simulink model "Avionics"  (R2022b)
settings: Solver=VariableStepAuto  StartTime=0.0  StopTime=10.0  RelTol=1e-3
settings Model: Creator=amira  LastModifiedBy=amira

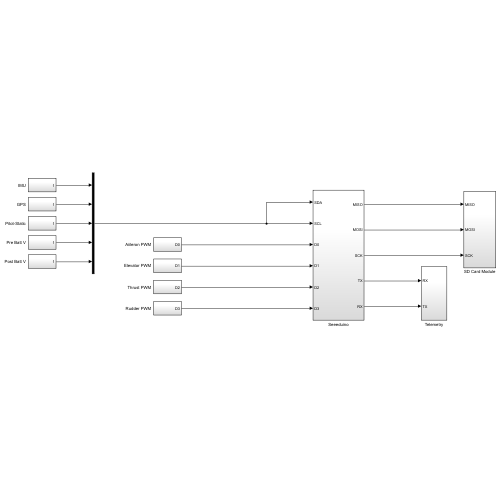
[thumbnail: Simulink's stored preview of the top-level diagram]
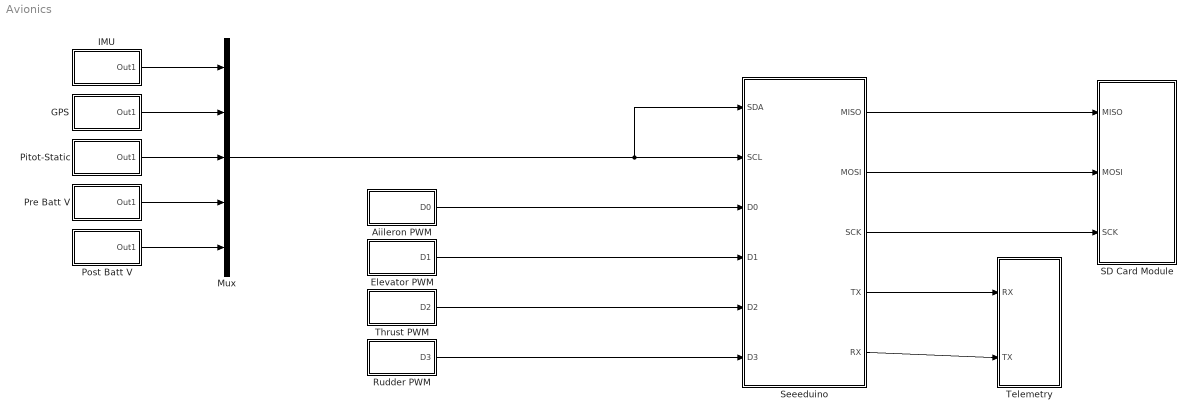
== system Avionics ==
  Aiileron PWM : Subsystem
  Elevator PWM : Subsystem
  GPS : Subsystem
  IMU : Subsystem
  Mux : Mux  Inputs=5
  Pitot-Static : Subsystem
  Post Batt V : Subsystem
  Pre Batt V : Subsystem
  Rudder PWM : Subsystem
  SD Card Module : Subsystem
  Seeeduino : Subsystem
  Telemetry : Subsystem
  Thrust PWM : Subsystem
  wires:
  Pitot-Static/1(Out1) -> Mux/3
  GPS/1(Out1) -> Mux/2
  IMU/1(Out1) -> Mux/1
  Pre Batt V/1(Out1) -> Mux/4
  Post Batt V/1(Out1) -> Mux/5
  Mux/1 -> Seeeduino/1(SDA), Seeeduino/2(SCL)
  Rudder PWM/1(D3) -> Seeeduino/6(D3)
  Thrust PWM/1(D2) -> Seeeduino/5(D2)
  Aiileron PWM/1(D0) -> Seeeduino/3(D0)
  Elevator PWM/1(D1) -> Seeeduino/4(D1)
  Seeeduino/1(MISO) -> SD Card Module/1(MISO)
  Seeeduino/2(MOSI) -> SD Card Module/2(MOSI)
  Seeeduino/3(SCK) -> SD Card Module/3(SCK)
  Seeeduino/4(TX) -> Telemetry/1(RX)
  Seeeduino/5(RX) -> Telemetry/2(TX)

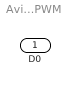
== system Avionics/Aiileron PWM ==
  D0 : Outport

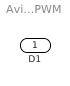
== system Avionics/Elevator PWM ==
  D1 : Outport

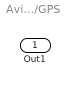
== system Avionics/GPS ==
  Out1 : Outport

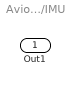
== system Avionics/IMU ==
  Out1 : Outport

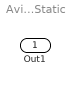
== system Avionics/Pitot-Static ==
  Out1 : Outport

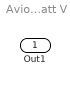
== system Avionics/Post Batt V ==
  Out1 : Outport

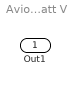
== system Avionics/Pre Batt V ==
  Out1 : Outport

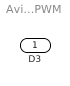
== system Avionics/Rudder PWM ==
  D3 : Outport

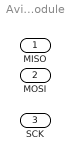
== system Avionics/SD Card Module ==
  MISO : Inport
  MOSI : Inport  Port=2
  SCK : Inport  Port=3

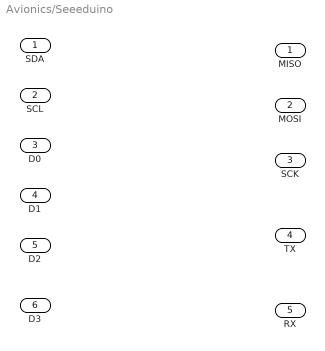
== system Avionics/Seeeduino ==
  SDA : Inport
  SCL : Inport  Port=2
  D0 : Inport  Port=3
  D1 : Inport  Port=4
  D2 : Inport  Port=5
  D3 : Inport  Port=6
  MISO : Outport
  MOSI : Outport  Port=2
  SCK : Outport  Port=3
  TX : Outport  Port=4
  RX : Outport  Port=5

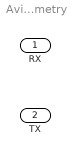
== system Avionics/Telemetry ==
  RX : Inport
  TX : Inport  Port=2

== system Avionics/Thrust PWM ==
  D2 : Outport
